simulink library "ssc_Probes_2012a_org"  (Simulink 10.0)
settings: Solver=ode45  StartTime=0.0  StopTime=10.0  RelTol=1e-3  EnableMultiTasking=on
libraries: fl_lib x42, nesl_utility x31, fl_ps_legacy_lib x1
(part 1 of 2)
settings Model: Creator=tegel  LastModifiedBy=bhisma

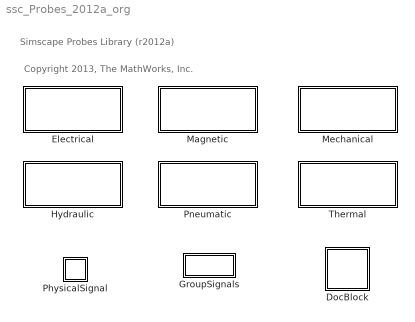
== system ssc_Probes_2012a_org ==
  note: Simscape Probes Library (r2012a)
  note: Copyright 2013, The MathWorks, Inc.
  DocBlock : Subsystem  mask(DocBlock){ECoderFlag=, DocumentType=Text}
      mask prompts: ECoderFlag "RTW Embedded Coder Flag"; DocumentType "Document Type"
      mask help: Use this block to save long descriptive text with the model. Double-clicking the block will open an editor.
      settings: DeleteFcn=docblock('close_document',gcb);  PreSaveFcn=docblock('save_document',gcb);  OpenFcn=docblock('edit_document',gcb);
      mask TypeOptions DocumentType: Text | RTF | HTML
      mask Display: disp('Help')
  Electrical : Subsystem
      mask Display: disp('Electrical')
  GroupSignals : Subsystem
      settings: OpenFcn=GroupSignals
      settings: CopyFcn=|
      | set_param(gcb,'LinkStatus','inactive')
      | set_param(gcb,'LinkStatus','none')
      mask Display: disp('Select')
  Hydraulic : Subsystem
      mask Display: disp('Hydraulic')
  Magnetic : Subsystem
      mask Display: disp('Magnetic');
  Mechanical : Subsystem
      mask Display: disp('Mechanical');
  PhysicalSignal : Subsystem  Description=Simscape Probe  InitFcn=|  StopFcn=|
      InitFcn=|
      | unit=get_param([gcb '/PS-S'],'Unit');                                              
      | set_param(gcb, 'AttributesFormatString', strcat('[', unit,']'));
      StopFcn=|
      | % Convert logsout to Dataset                                
      | if ~strcmp(class(logsout),'Simulink.SimulationData.Dataset')
      | logsout = logsout.convertToDataset('logsout');              
      | end
      mask help: Simscape Probe
      settings: CopyFcn=|
      | set_param(gcb,'LinkStatus','inactive');
      | set_param(gcb,'LinkStatus','none');
      | set_param([gcb '/Goto'],'GotoTag', [get(gcbh,'name')]);
      | set_param([gcb '/From'],'GotoTag', [get(gcbh,'name')]);
      | h = get_param([gcb, '/PS-S'], 'PortHandles');
      | set(h.Outport(1), 'SignalNameFromLabel', [get(gcbh,'name')])
      | clear h;
      settings: NameChangeFcn=|
      | set_param([gcb '/Goto'],'GotoTag', [get(gcbh,'name')]);
      | set_param([gcb '/From'],'GotoTag', [get(gcbh,'name')]);
      | h = get_param([gcb, '/PS-S'], 'PortHandles');
      | set(h.Outport(1), 'SignalNameFromLabel', [get(gcbh,'name')])
      | clear h;
      settings: OpenFcn=|
      | if exist('logsout', 'var')
      |   vname = get(gcbh,'name');
      |   fHandle = findall(0,'Tag',vname);
      |   if isempty(fHandle)
      |   figure('Tag',vname);
      |   end;
      |   figure(findobj('Tag',vname));
      |   plot(logsout.getElement([gcb, '/PS-S'], '-blockpath').Values)
      |   title(get(gcbh,'name'));
      |   ylabel(['Physical Signal (' get_param([gcb '/PS-S'],'Unit') ')'] );
      | end
      mask Display: disp('PS');
  Pneumatic : Subsystem
      mask Display: disp('Pneumatic');
  Thermal : Subsystem
      mask Display: disp('Thermal');

== system ssc_Probes_2012a_org/DocBlock ==
  EmptySubsystem : Subsystem

== system ssc_Probes_2012a_org/Electrical ==
  note: Electrical Probes
  note: Across Variable
      | (Internal Reference)
  note: Through
      | Variable
  note: Across Variable
      | (Differential)
  Current : Subsystem  Description=Simscape Probe  InitFcn=|  StopFcn=|
      InitFcn=|
      | unit=get_param([gcb '/PS-S'],'Unit');                                              
      | set_param(gcb, 'AttributesFormatString', strcat('[', unit,']'));
      StopFcn=|
      | % Convert logsout to Dataset                                
      | if ~strcmp(class(logsout),'Simulink.SimulationData.Dataset')
      | logsout = logsout.convertToDataset('logsout');              
      | end
      mask help: Simscape Probe
      settings: CopyFcn=|
      | set_param(gcb,'LinkStatus','inactive');
      | set_param(gcb,'LinkStatus','none');
      | set_param([gcb '/Goto'],'GotoTag', [get(gcbh,'name')]);
      | set_param([gcb '/From'],'GotoTag', [get(gcbh,'name')]);
      | h = get_param([gcb, '/PS-S'], 'PortHandles');
      | set(h.Outport(1), 'SignalNameFromLabel', [get(gcbh,'name')])
      | clear h;
      settings: NameChangeFcn=|
      | set_param([gcb '/Goto'],'GotoTag', [get(gcbh,'name')]);
      | set_param([gcb '/From'],'GotoTag', [get(gcbh,'name')]);
      | h = get_param([gcb, '/PS-S'], 'PortHandles');
      | set(h.Outport(1), 'SignalNameFromLabel', [get(gcbh,'name')])
      | clear h;
      settings: OpenFcn=|
      | if exist('logsout', 'var')
      |   vname = get(gcbh,'name');
      |   fHandle = findall(0,'Tag',vname);
      |   if isempty(fHandle)
      |   figure('Tag',vname);
      |   end;
      |   figure(findobj('Tag',vname));
      |   plot(logsout.getElement([gcb, '/PS-S'], '-blockpath').Values)
      |   title(get(gcbh,'name'));
      |   ylabel(['Current (' get_param([gcb '/PS-S'],'Unit') ')'] );
      | end
      mask Display:
      | patch([0.5 1 0.5], [0.25 .5 0.75],[0.7 0.7 0.7])
      | plot([0,0.5],[0.5,0.5]);
  Voltage : Subsystem  Description=Simscape Probe  InitFcn=|  StopFcn=|
      InitFcn=|
      | unit=get_param([gcb '/PS-S'],'Unit');                                              
      | set_param(gcb, 'AttributesFormatString', strcat('[', unit,']'));
      StopFcn=|
      | % Convert logsout to Dataset                                
      | if ~strcmp(class(logsout),'Simulink.SimulationData.Dataset')
      | logsout = logsout.convertToDataset('logsout');              
      | end
      mask help: Simscape Probe
      settings: CopyFcn=|
      | set_param(gcb,'LinkStatus','inactive');
      | set_param(gcb,'LinkStatus','none');
      | set_param([gcb '/Goto'],'GotoTag', [get(gcbh,'name')]);
      | set_param([gcb '/From'],'GotoTag', [get(gcbh,'name')]);
      | h = get_param([gcb, '/PS-S'], 'PortHandles');
      | set(h.Outport(1), 'SignalNameFromLabel', [get(gcbh,'name')])
      | clear h;
      settings: NameChangeFcn=|
      | set_param([gcb '/Goto'],'GotoTag', [get(gcbh,'name')]);
      | set_param([gcb '/From'],'GotoTag', [get(gcbh,'name')]);
      | h = get_param([gcb, '/PS-S'], 'PortHandles');
      | set(h.Outport(1), 'SignalNameFromLabel', [get(gcbh,'name')])
      | clear h;
      settings: OpenFcn=|
      | if exist('logsout', 'var')
      |   vname = get(gcbh,'name');
      |   fHandle = findall(0,'Tag',vname);
      |   if isempty(fHandle)
      |   figure('Tag',vname);
      |   end;
      |   figure(findobj('Tag',vname));
      |   plot(logsout.getElement([gcb, '/PS-S'], '-blockpath').Values)
      |   title(get(gcbh,'name'));
      |   ylabel(['Voltage (' get_param([gcb '/PS-S'],'Unit') ')'] );
      | end
      mask Display: port_label('LConn', 1,'V');
  dVoltage : Subsystem  Description=Simscape Probe  InitFcn=|  StopFcn=|
      InitFcn=|
      | unit=get_param([gcb '/PS-S'],'Unit');                                              
      | set_param(gcb, 'AttributesFormatString', strcat('[', unit,']'));
      StopFcn=|
      | % Convert logsout to Dataset                                
      | if ~strcmp(class(logsout),'Simulink.SimulationData.Dataset')
      | logsout = logsout.convertToDataset('logsout');              
      | end
      mask help: Simscape Probe
      settings: CopyFcn=|
      | set_param(gcb,'LinkStatus','inactive');
      | set_param(gcb,'LinkStatus','none');
      | set_param([gcb '/Goto'],'GotoTag', [get(gcbh,'name')]);
      | set_param([gcb '/From'],'GotoTag', [get(gcbh,'name')]);
      | h = get_param([gcb, '/PS-S'], 'PortHandles');
      | set(h.Outport(1), 'SignalNameFromLabel', [get(gcbh,'name')])
      | clear h;
      settings: NameChangeFcn=|
      | set_param([gcb '/Goto'],'GotoTag', [get(gcbh,'name')]);
      | set_param([gcb '/From'],'GotoTag', [get(gcbh,'name')]);
      | h = get_param([gcb, '/PS-S'], 'PortHandles');
      | set(h.Outport(1), 'SignalNameFromLabel', [get(gcbh,'name')])
      | clear h;
      settings: OpenFcn=|
      | if exist('logsout', 'var')
      |   vname = get(gcbh,'name');
      |   fHandle = findall(0,'Tag',vname);
      |   if isempty(fHandle)
      |   figure('Tag',vname);
      |   end;
      |   figure(findobj('Tag',vname));
      |   plot(logsout.getElement([gcb, '/PS-S'], '-blockpath').Values)
      |   title(get(gcbh,'name'));
      |   ylabel(['Voltage (' get_param([gcb '/PS-S'],'Unit') ')'] );
      | end
      mask Display:
      | port_label('RConn', 1,'-');
      | port_label('LConn', 1,'+');

== system ssc_Probes_2012a_org/GroupSignals ==

== system ssc_Probes_2012a_org/Hydraulic ==
  note: Hydraulic Probes
  note: Across Variable
      | (Internal Reference)
  note: Through
      | Variable
  note: Across Variable
      | (Differential)
  Flow : Subsystem  Description=Simscape Probe  InitFcn=|  StopFcn=|
      InitFcn=|
      | unit=get_param([gcb '/PS-S'],'Unit');                                              
      | set_param(gcb, 'AttributesFormatString', strcat('[', unit,']'));
      StopFcn=|
      | % Convert logsout to Dataset                                
      | if ~strcmp(class(logsout),'Simulink.SimulationData.Dataset')
      | logsout = logsout.convertToDataset('logsout');              
      | end
      mask help: Simscape Probe
      settings: CopyFcn=|
      | set_param(gcb,'LinkStatus','inactive');
      | set_param(gcb,'LinkStatus','none');
      | set_param([gcb '/Goto'],'GotoTag', [get(gcbh,'name')]);
      | set_param([gcb '/From'],'GotoTag', [get(gcbh,'name')]);
      | h = get_param([gcb, '/PS-S'], 'PortHandles');
      | set(h.Outport(1), 'SignalNameFromLabel', [get(gcbh,'name')])
      | clear h;
      settings: NameChangeFcn=|
      | set_param([gcb '/Goto'],'GotoTag', [get(gcbh,'name')]);
      | set_param([gcb '/From'],'GotoTag', [get(gcbh,'name')]);
      | h = get_param([gcb, '/PS-S'], 'PortHandles');
      | set(h.Outport(1), 'SignalNameFromLabel', [get(gcbh,'name')])
      | clear h;
      settings: OpenFcn=|
      | if exist('logsout', 'var')
      |   vname = get(gcbh,'name');
      |   fHandle = findall(0,'Tag',vname);
      |   if isempty(fHandle)
      |   figure('Tag',vname);
      |   end;
      |   figure(findobj('Tag',vname));
      |   plot(logsout.getElement([gcb, '/PS-S'], '-blockpath').Values)
      |   title(get(gcbh,'name'));
      |   ylabel(['Flow (' get_param([gcb '/PS-S'],'Unit') ')'] );
      | end
      mask Display:
      | patch([0.5 1 0.5], [0.25 .5 0.75],[0.7 0.7 0.7])
      | plot([0,0.5],[0.5,0.5]);
  Pressure : Subsystem  Description=Simscape Probe  InitFcn=|  StopFcn=|
      InitFcn=|
      | unit=get_param([gcb '/PS-S'],'Unit');                                              
      | set_param(gcb, 'AttributesFormatString', strcat('[', unit,']'));
      StopFcn=|
      | % Convert logsout to Dataset                                
      | if ~strcmp(class(logsout),'Simulink.SimulationData.Dataset')
      | logsout = logsout.convertToDataset('logsout');              
      | end
      mask help: Simscape Probe
      settings: CopyFcn=|
      | set_param(gcb,'LinkStatus','inactive');
      | set_param(gcb,'LinkStatus','none');
      | set_param([gcb '/Goto'],'GotoTag', [get(gcbh,'name')]);
      | set_param([gcb '/From'],'GotoTag', [get(gcbh,'name')]);
      | h = get_param([gcb, '/PS-S'], 'PortHandles');
      | set(h.Outport(1), 'SignalNameFromLabel', [get(gcbh,'name')])
      | clear h;
      settings: NameChangeFcn=|
      | set_param([gcb '/Goto'],'GotoTag', [get(gcbh,'name')]);
      | set_param([gcb '/From'],'GotoTag', [get(gcbh,'name')]);
      | h = get_param([gcb, '/PS-S'], 'PortHandles');
      | set(h.Outport(1), 'SignalNameFromLabel', [get(gcbh,'name')])
      | clear h;
      settings: OpenFcn=|
      | if exist('logsout', 'var')
      |   vname = get(gcbh,'name');
      |   fHandle = findall(0,'Tag',vname);
      |   if isempty(fHandle)
      |   figure('Tag',vname);
      |   end;
      |   figure(findobj('Tag',vname));
      |   plot(logsout.getElement([gcb, '/PS-S'], '-blockpath').Values)
      |   title(get(gcbh,'name'));
      |   ylabel(['Pressure (' get_param([gcb '/PS-S'],'Unit') ')'] );
      | end
      mask Display: port_label('LConn', 1,'P');
  dPressure : Subsystem  Description=Simscape Probe  InitFcn=|  StopFcn=|
      InitFcn=|
      | unit=get_param([gcb '/PS-S'],'Unit');                                             
      | set_param(gcb, 'AttributesFormatString', strcat('[', unit,']'));
      StopFcn=|
      | % Convert logsout to Dataset                                
      | if ~strcmp(class(logsout),'Simulink.SimulationData.Dataset')
      | logsout = logsout.convertToDataset('logsout');              
      | end
      mask help: Simscape Probe
      settings: CopyFcn=|
      | set_param(gcb,'LinkStatus','inactive');
      | set_param(gcb,'LinkStatus','none');
      | set_param([gcb '/Goto'],'GotoTag', [get(gcbh,'name')]);
      | set_param([gcb '/From'],'GotoTag', [get(gcbh,'name')]);
      | h = get_param([gcb, '/PS-S'], 'PortHandles');
      | set(h.Outport(1), 'SignalNameFromLabel', [get(gcbh,'name')])
      | clear h;
      settings: NameChangeFcn=|
      | set_param([gcb '/Goto'],'GotoTag', [get(gcbh,'name')]);
      | set_param([gcb '/From'],'GotoTag', [get(gcbh,'name')]);
      | h = get_param([gcb, '/PS-S'], 'PortHandles');
      | set(h.Outport(1), 'SignalNameFromLabel', [get(gcbh,'name')])
      | clear h;
      settings: OpenFcn=|
      | if exist('logsout', 'var')
      |   vname = get(gcbh,'name');
      |   fHandle = findall(0,'Tag',vname);
      |   if isempty(fHandle)
      |   figure('Tag',vname);
      |   end;
      |   figure(findobj('Tag',vname));
      |   plot(logsout.getElement([gcb, '/PS-S'], '-blockpath').Values)
      |   title(get(gcbh,'name'));
      |   ylabel(['Pressure (' get_param([gcb '/PS-S'],'Unit') ')'] );
      | end
      mask Display:
      | port_label('RConn', 1,'-');
      | port_label('LConn', 1,'+');

== system ssc_Probes_2012a_org/Magnetic ==
  note: Across Variable
      | (Differential)
  note: Through
      | Variable
  note: Across Variable
      | (Internal Reference)
  note: MagneticProbes
  Flux : Subsystem  Description=Simscape Probe  InitFcn=|  StopFcn=|
      InitFcn=|
      | unit=get_param([gcb '/PS-S'],'Unit');                                              
      | set_param(gcb, 'AttributesFormatString', strcat('[', unit,']'));
      StopFcn=|
      | % Convert logsout to Dataset                                
      | if ~strcmp(class(logsout),'Simulink.SimulationData.Dataset')
      | logsout = logsout.convertToDataset('logsout');              
      | end
      mask help: Simscape Probe
      settings: CopyFcn=|
      | set_param(gcb,'LinkStatus','inactive');
      | set_param(gcb,'LinkStatus','none');
      | set_param([gcb '/Goto'],'GotoTag', [get(gcbh,'name')]);
      | set_param([gcb '/From'],'GotoTag', [get(gcbh,'name')]);
      | h = get_param([gcb, '/PS-S'], 'PortHandles');
      | set(h.Outport(1), 'SignalNameFromLabel', [get(gcbh,'name')])
      | clear h;
      settings: NameChangeFcn=|
      | set_param([gcb '/Goto'],'GotoTag', [get(gcbh,'name')]);
      | set_param([gcb '/From'],'GotoTag', [get(gcbh,'name')]);
      | h = get_param([gcb, '/PS-S'], 'PortHandles');
      | set(h.Outport(1), 'SignalNameFromLabel', [get(gcbh,'name')])
      | clear h;
      settings: OpenFcn=|
      | if exist('logsout', 'var')
      |   vname = get(gcbh,'name');
      |   fHandle = findall(0,'Tag',vname);
      |   if isempty(fHandle)
      |   figure('Tag',vname);
      |   end;
      |   figure(findobj('Tag',vname));
      |   plot(logsout.getElement([gcb, '/PS-S'], '-blockpath').Values)
      |   title(get(gcbh,'name'));
      |   ylabel(['Flux (' get_param([gcb '/PS-S'],'Unit') ')'] );
      | end
      mask Display:
      | patch([0.5 1 0.5], [0.25 .5 0.75],[0.7 0.7 0.7])
      | plot([0,0.5],[0.5,0.5]);
  MMF : Subsystem  Description=Simscape Probe  InitFcn=|  StopFcn=|
      InitFcn=|
      | unit=get_param([gcb '/PS-S'],'Unit');                                              
      | set_param(gcb, 'AttributesFormatString', strcat('[', unit,']'));
      StopFcn=|
      | % Convert logsout to Dataset                                
      | if ~strcmp(class(logsout),'Simulink.SimulationData.Dataset')
      | logsout = logsout.convertToDataset('logsout');              
      | end
      mask help: Simscape Probe
      settings: CopyFcn=|
      | set_param(gcb,'LinkStatus','inactive');
      | set_param(gcb,'LinkStatus','none');
      | set_param([gcb '/Goto'],'GotoTag', [get(gcbh,'name')]);
      | set_param([gcb '/From'],'GotoTag', [get(gcbh,'name')]);
      | h = get_param([gcb, '/PS-S'], 'PortHandles');
      | set(h.Outport(1), 'SignalNameFromLabel', [get(gcbh,'name')])
      | clear h;
      settings: NameChangeFcn=|
      | set_param([gcb '/Goto'],'GotoTag', [get(gcbh,'name')]);
      | set_param([gcb '/From'],'GotoTag', [get(gcbh,'name')]);
      | h = get_param([gcb, '/PS-S'], 'PortHandles');
      | set(h.Outport(1), 'SignalNameFromLabel', [get(gcbh,'name')])
      | clear h;
      settings: OpenFcn=|
      | if exist('logsout', 'var')
      |   vname = get(gcbh,'name');
      |   fHandle = findall(0,'Tag',vname);
      |   if isempty(fHandle)
      |   figure('Tag',vname);
      |   end;
      |   figure(findobj('Tag',vname));
      |   plot(logsout.getElement([gcb, '/PS-S'], '-blockpath').Values)
      |   title(get(gcbh,'name'));
      |   ylabel(['MMF (' get_param([gcb '/PS-S'],'Unit') ')'] );
      | end
      mask Display: port_label('LConn', 1,'F');
  dMMF : Subsystem  Description=Simscape Probe  InitFcn=|  StopFcn=|
      InitFcn=|
      | unit=get_param([gcb '/PS-S'],'Unit');                                              
      | set_param(gcb, 'AttributesFormatString', strcat('[', unit,']'));
      StopFcn=|
      | % Convert logsout to Dataset                                
      | if ~strcmp(class(logsout),'Simulink.SimulationData.Dataset')
      | logsout = logsout.convertToDataset('logsout');              
      | end
      mask help: Simscape Probe
      settings: CopyFcn=|
      | set_param(gcb,'LinkStatus','inactive');
      | set_param(gcb,'LinkStatus','none');
      | set_param([gcb '/Goto'],'GotoTag', [get(gcbh,'name')]);
      | set_param([gcb '/From'],'GotoTag', [get(gcbh,'name')]);
      | h = get_param([gcb, '/PS-S'], 'PortHandles');
      | set(h.Outport(1), 'SignalNameFromLabel', [get(gcbh,'name')])
      | clear h;
      settings: NameChangeFcn=|
      | set_param([gcb '/Goto'],'GotoTag', [get(gcbh,'name')]);
      | set_param([gcb '/From'],'GotoTag', [get(gcbh,'name')]);
      | h = get_param([gcb, '/PS-S'], 'PortHandles');
      | set(h.Outport(1), 'SignalNameFromLabel', [get(gcbh,'name')])
      | clear h;
      settings: OpenFcn=|
      | if exist('logsout', 'var')
      |   vname = get(gcbh,'name');
      |   fHandle = findall(0,'Tag',vname);
      |   if isempty(fHandle)
      |   figure('Tag',vname);
      |   end;
      |   figure(findobj('Tag',vname));
      |   plot(logsout.getElement([gcb, '/PS-S'], '-blockpath').Values)
      |   title(get(gcbh,'name'));
      |   ylabel(['MMF (' get_param([gcb '/PS-S'],'Unit') ')'] );
      | end
      mask Display:
      | port_label('RConn', 1,'-');
      | port_label('LConn', 1,'+');

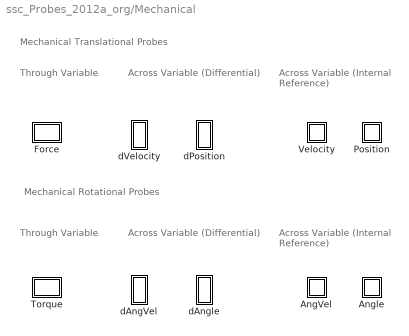
== system ssc_Probes_2012a_org/Mechanical ==
  note: Across Variable
      | (Differential)
  note: Through
      | Variable
  note: Across Variable
      | (Internal Reference)
  note: Mechanical Translational Probes
  note: Across Variable
      | (Differential)
  note: Through
      | Variable
  note: Across Variable
      | (Internal Reference)
  note: Mechanical Rotational Probes
  AngVel : Subsystem  Description=Simscape Probe  InitFcn=|  StopFcn=|
      InitFcn=|
      | unit=get_param([gcb '/PS-S'],'Unit');                                              
      | set_param(gcb, 'AttributesFormatString', strcat('[', unit,']'));
      StopFcn=|
      | % Convert logsout to Dataset                                
      | if ~strcmp(class(logsout),'Simulink.SimulationData.Dataset')
      | logsout = logsout.convertToDataset('logsout');              
      | end
      mask help: Simscape Probe
      settings: CopyFcn=|
      | set_param(gcb,'LinkStatus','inactive');
      | set_param(gcb,'LinkStatus','none');
      | set_param([gcb '/Goto'],'GotoTag', [get(gcbh,'name')]);
      | set_param([gcb '/From'],'GotoTag', [get(gcbh,'name')]);
      | h = get_param([gcb, '/PS-S'], 'PortHandles');
      | set(h.Outport(1), 'SignalNameFromLabel', [get(gcbh,'name')])
      | clear h;
      settings: NameChangeFcn=|
      | set_param([gcb '/Goto'],'GotoTag', [get(gcbh,'name')]);
      | set_param([gcb '/From'],'GotoTag', [get(gcbh,'name')]);
      | h = get_param([gcb, '/PS-S'], 'PortHandles');
      | set(h.Outport(1), 'SignalNameFromLabel', [get(gcbh,'name')])
      | clear h;
      settings: OpenFcn=|
      | if exist('logsout', 'var')
      |   vname = get(gcbh,'name');
      |   fHandle = findall(0,'Tag',vname);
      |   if isempty(fHandle)
      |   figure('Tag',vname);
      |   end;
      |   figure(findobj('Tag',vname));
      |   plot(logsout.getElement([gcb, '/PS-S'], '-blockpath').Values)
      |   title(get(gcbh,'name'));
      |   ylabel(['Anguiar Velocity (' get_param([gcb '/PS-S'],'Unit') ')'] );
      | end
      mask Display: port_label('LConn', 1,'W');
  Angle : Subsystem  Description=Simscape Probe  InitFcn=|  StopFcn=|
      InitFcn=|
      | unit=get_param([gcb '/PS-S'],'Unit');                                              
      | set_param(gcb, 'AttributesFormatString', strcat('[', unit,']'));
      StopFcn=|
      | % Convert logsout to Dataset                                
      | if ~strcmp(class(logsout),'Simulink.SimulationData.Dataset')
      | logsout = logsout.convertToDataset('logsout');              
      | end
      mask help: Simscape Probe
      settings: CopyFcn=|
      | set_param(gcb,'LinkStatus','inactive');
      | set_param(gcb,'LinkStatus','none');
      | set_param([gcb '/Goto'],'GotoTag', [get(gcbh,'name')]);
      | set_param([gcb '/From'],'GotoTag', [get(gcbh,'name')]);
      | h = get_param([gcb, '/PS-S'], 'PortHandles');
      | set(h.Outport(1), 'SignalNameFromLabel', [get(gcbh,'name')])
      | clear h;
      settings: NameChangeFcn=|
      | set_param([gcb '/Goto'],'GotoTag', [get(gcbh,'name')]);
      | set_param([gcb '/From'],'GotoTag', [get(gcbh,'name')]);
      | h = get_param([gcb, '/PS-S'], 'PortHandles');
      | set(h.Outport(1), 'SignalNameFromLabel', [get(gcbh,'name')])
      | clear h;
      settings: OpenFcn=|
      | if exist('logsout', 'var')
      |   vname = get(gcbh,'name');
      |   fHandle = findall(0,'Tag',vname);
      |   if isempty(fHandle)
      |   figure('Tag',vname);
      |   end;
      |   figure(findobj('Tag',vname));
      |   plot(logsout.getElement([gcb, '/PS-S'], '-blockpath').Values)
      |   title(get(gcbh,'name'));
      |   ylabel(['Angle (' get_param([gcb '/PS-S'],'Unit') ')'] );
      | end
      mask Display: port_label('LConn', 1,'A');
  Force : Subsystem  Description=Simscape Probe  InitFcn=|  StopFcn=|
      InitFcn=|
      | unit=get_param([gcb '/PS-S'],'Unit');                                              
      | set_param(gcb, 'AttributesFormatString', strcat('[', unit,']'));
      StopFcn=|
      | % Convert logsout to Dataset                                
      | if ~strcmp(class(logsout),'Simulink.SimulationData.Dataset')
      | logsout = logsout.convertToDataset('logsout');              
      | end
      mask help: Simscape Probe
      settings: CopyFcn=|
      | set_param(gcb,'LinkStatus','inactive');
      | set_param(gcb,'LinkStatus','none');
      | set_param([gcb '/Goto'],'GotoTag', [get(gcbh,'name')]);
      | set_param([gcb '/From'],'GotoTag', [get(gcbh,'name')]);
      | h = get_param([gcb, '/PS-S'], 'PortHandles');
      | set(h.Outport(1), 'SignalNameFromLabel', [get(gcbh,'name')])
      | clear h;
      settings: NameChangeFcn=|
      | set_param([gcb '/Goto'],'GotoTag', [get(gcbh,'name')]);
      | set_param([gcb '/From'],'GotoTag', [get(gcbh,'name')]);
      | h = get_param([gcb, '/PS-S'], 'PortHandles');
      | set(h.Outport(1), 'SignalNameFromLabel', [get(gcbh,'name')])
      | clear h;
      settings: OpenFcn=|
      | if exist('logsout', 'var')
      |   vname = get(gcbh,'name');
      |   fHandle = findall(0,'Tag',vname);
      |   if isempty(fHandle)
      |   figure('Tag',vname);
      |   end;
      |   figure(findobj('Tag',vname));
      |   plot(logsout.getElement([gcb, '/PS-S'], '-blockpath').Values)
      |   title(get(gcbh,'name'));
      |   ylabel(['Force (' get_param([gcb '/PS-S'],'Unit') ')'] );
      | end
      mask Display:
      | patch([0.5 1 0.5], [0.25 .5 0.75],[0.7 0.7 0.7])
      | plot([0,0.5],[0.5,0.5]);
  Position : Subsystem  Description=Simscape Probe  InitFcn=|  StopFcn=|
      InitFcn=|
      | unit=get_param([gcb '/PS-S'],'Unit');                                              
      | set_param(gcb, 'AttributesFormatString', strcat('[', unit,']'));
      StopFcn=|
      | % Convert logsout to Dataset                                
      | if ~strcmp(class(logsout),'Simulink.SimulationData.Dataset')
      | logsout = logsout.convertToDataset('logsout');              
      | end
      mask help: Simscape Probe
      settings: CopyFcn=|
      | set_param(gcb,'LinkStatus','inactive');
      | set_param(gcb,'LinkStatus','none');
      | set_param([gcb '/Goto'],'GotoTag', [get(gcbh,'name')]);
      | set_param([gcb '/From'],'GotoTag', [get(gcbh,'name')]);
      | h = get_param([gcb, '/PS-S'], 'PortHandles');
      | set(h.Outport(1), 'SignalNameFromLabel', [get(gcbh,'name')])
      | clear h;
      settings: NameChangeFcn=|
      | set_param([gcb '/Goto'],'GotoTag', [get(gcbh,'name')]);
      | set_param([gcb '/From'],'GotoTag', [get(gcbh,'name')]);
      | h = get_param([gcb, '/PS-S'], 'PortHandles');
      | set(h.Outport(1), 'SignalNameFromLabel', [get(gcbh,'name')])
      | clear h;
      settings: OpenFcn=|
      | if exist('logsout', 'var')
      |   vname = get(gcbh,'name');
      |   fHandle = findall(0,'Tag',vname);
      |   if isempty(fHandle)
      |   figure('Tag',vname);
      |   end;
      |   figure(findobj('Tag',vname));
      |   plot(logsout.getElement([gcb, '/PS-S'], '-blockpath').Values)
      |   title(get(gcbh,'name'));
      |   ylabel(['Position (' get_param([gcb '/PS-S'],'Unit') ')'] );
      | end
      mask Display: port_label('LConn', 1,'P');
  Torque : Subsystem  Description=Simscape Probe  InitFcn=|  StopFcn=|
      InitFcn=|
      | unit=get_param([gcb '/PS-S'],'Unit');                                              
      | set_param(gcb, 'AttributesFormatString', strcat('[', unit,']'));
      StopFcn=|
      | % Convert logsout to Dataset                                
      | if ~strcmp(class(logsout),'Simulink.SimulationData.Dataset')
      | logsout = logsout.convertToDataset('logsout');              
      | end
      mask help: Simscape Probe
      settings: CopyFcn=|
      | set_param(gcb,'LinkStatus','inactive');
      | set_param(gcb,'LinkStatus','none');
      | set_param([gcb '/Goto'],'GotoTag', [get(gcbh,'name')]);
      | set_param([gcb '/From'],'GotoTag', [get(gcbh,'name')]);
      | h = get_param([gcb, '/PS-S'], 'PortHandles');
      | set(h.Outport(1), 'SignalNameFromLabel', [get(gcbh,'name')])
      | clear h;
      settings: NameChangeFcn=|
      | set_param([gcb '/Goto'],'GotoTag', [get(gcbh,'name')]);
      | set_param([gcb '/From'],'GotoTag', [get(gcbh,'name')]);
      | h = get_param([gcb, '/PS-S'], 'PortHandles');
      | set(h.Outport(1), 'SignalNameFromLabel', [get(gcbh,'name')])
      | clear h;
      settings: OpenFcn=|
      | if exist('logsout', 'var')
      |   vname = get(gcbh,'name');
      |   fHandle = findall(0,'Tag',vname);
      |   if isempty(fHandle)
      |   figure('Tag',vname);
      |   end;
      |   figure(findobj('Tag',vname));
      |   plot(logsout.getElement([gcb, '/PS-S'], '-blockpath').Values)
      |   title(get(gcbh,'name'));
      |   ylabel(['Torque (' get_param([gcb '/PS-S'],'Unit') ')'] );
      | end
      mask Display:
      | patch([0.5 1 0.5], [0.25 .5 0.75],[0.7 0.7 0.7])
      | plot([0,0.5],[0.5,0.5]);
  Velocity : Subsystem  Description=Simscape Probe  InitFcn=|  StopFcn=|
      InitFcn=|
      | unit=get_param([gcb '/PS-S'],'Unit');                                              
      | set_param(gcb, 'AttributesFormatString', strcat('[', unit,']'));
      StopFcn=|
      | % Convert logsout to Dataset                                
      | if ~strcmp(class(logsout),'Simulink.SimulationData.Dataset')
      | logsout = logsout.convertToDataset('logsout');              
      | end
      mask help: Simscape Probe
      settings: CopyFcn=|
      | set_param(gcb,'LinkStatus','inactive');
      | set_param(gcb,'LinkStatus','none');
      | set_param([gcb '/Goto'],'GotoTag', [get(gcbh,'name')]);
      | set_param([gcb '/From'],'GotoTag', [get(gcbh,'name')]);
      | h = get_param([gcb, '/PS-S'], 'PortHandles');
      | set(h.Outport(1), 'SignalNameFromLabel', [get(gcbh,'name')])
      | clear h;
      settings: NameChangeFcn=|
      | set_param([gcb '/Goto'],'GotoTag', [get(gcbh,'name')]);
      | set_param([gcb '/From'],'GotoTag', [get(gcbh,'name')]);
      | h = get_param([gcb, '/PS-S'], 'PortHandles');
      | set(h.Outport(1), 'SignalNameFromLabel', [get(gcbh,'name')])
      | clear h;
      settings: OpenFcn=|
      | if exist('logsout', 'var')
      |   vname = get(gcbh,'name');
      |   fHandle = findall(0,'Tag',vname);
      |   if isempty(fHandle)
      |   figure('Tag',vname);
      |   end;
      |   figure(findobj('Tag',vname));
      |   plot(logsout.getElement([gcb, '/PS-S'], '-blockpath').Values)
      |   title(get(gcbh,'name'));
      |   ylabel(['Velocity (' get_param([gcb '/PS-S'],'Unit') ')'] );
      | end
      mask Display: port_label('LConn', 1,'V');
  dAngVel : Subsystem  Description=Simscape Probe  InitFcn=|  StopFcn=|
      InitFcn=|
      | unit=get_param([gcb '/PS-S'],'Unit');                                              
      | set_param(gcb, 'AttributesFormatString', strcat('[', unit,']'));
      StopFcn=|
      | % Convert logsout to Dataset                                
      | if ~strcmp(class(logsout),'Simulink.SimulationData.Dataset')
      | logsout = logsout.convertToDataset('logsout');              
      | end
      mask help: Simscape Probe
      settings: CopyFcn=|
      | set_param(gcb,'LinkStatus','inactive');
      | set_param(gcb,'LinkStatus','none');
      | set_param([gcb '/Goto'],'GotoTag', [get(gcbh,'name')]);
      | set_param([gcb '/From'],'GotoTag', [get(gcbh,'name')]);
      | h = get_param([gcb, '/PS-S'], 'PortHandles');
      | set(h.Outport(1), 'SignalNameFromLabel', [get(gcbh,'name')])
      | clear h;
      settings: NameChangeFcn=|
      | set_param([gcb '/Goto'],'GotoTag', [get(gcbh,'name')]);
      | set_param([gcb '/From'],'GotoTag', [get(gcbh,'name')]);
      | h = get_param([gcb, '/PS-S'], 'PortHandles');
      | set(h.Outport(1), 'SignalNameFromLabel', [get(gcbh,'name')])
      | clear h;
      settings: OpenFcn=|
      | if exist('logsout', 'var')
      |   vname = get(gcbh,'name');
      |   fHandle = findall(0,'Tag',vname);
      |   if isempty(fHandle)
      |   figure('Tag',vname);
      |   end;
      |   figure(findobj('Tag',vname));
      |   plot(logsout.getElement([gcb, '/PS-S'], '-blockpath').Values)
      |   title(get(gcbh,'name'));
      |   ylabel(['Angular Velocity (' get_param([gcb '/PS-S'],'Unit') ')'] );
      | end
      mask Display:
      | port_label('RConn', 1,'-');
      | port_label('LConn', 1,'+');
  dAngle : Subsystem  Description=Simscape Probe  InitFcn=|  StopFcn=|
      InitFcn=|
      | unit=get_param([gcb '/PS-S'],'Unit');                                              
      | set_param(gcb, 'AttributesFormatString', strcat('[', unit,']'));
      StopFcn=|
      | % Convert logsout to Dataset                                
      | if ~strcmp(class(logsout),'Simulink.SimulationData.Dataset')
      | logsout = logsout.convertToDataset('logsout');              
      | end
      mask help: Simscape Probe
      settings: CopyFcn=|
      | set_param(gcb,'LinkStatus','inactive');
      | set_param(gcb,'LinkStatus','none');
      | set_param([gcb '/Goto'],'GotoTag', [get(gcbh,'name')]);
      | set_param([gcb '/From'],'GotoTag', [get(gcbh,'name')]);
      | h = get_param([gcb, '/PS-S'], 'PortHandles');
      | set(h.Outport(1), 'SignalNameFromLabel', [get(gcbh,'name')])
      | clear h;
      settings: NameChangeFcn=|
      | set_param([gcb '/Goto'],'GotoTag', [get(gcbh,'name')]);
      | set_param([gcb '/From'],'GotoTag', [get(gcbh,'name')]);
      | h = get_param([gcb, '/PS-S'], 'PortHandles');
      | set(h.Outport(1), 'SignalNameFromLabel', [get(gcbh,'name')])
      | clear h;
      settings: OpenFcn=|
      | if exist('logsout', 'var')
      |   vname = get(gcbh,'name');
      |   fHandle = findall(0,'Tag',vname);
      |   if isempty(fHandle)
      |   figure('Tag',vname);
      |   end;
      |   figure(findobj('Tag',vname));
      |   plot(logsout.getElement([gcb, '/PS-S'], '-blockpath').Values)
      |   title(get(gcbh,'name'));
      |   ylabel(['Angle (' get_param([gcb '/PS-S'],'Unit') ')'] );
      | end
      mask Display:
      | port_label('RConn', 1,'-');
      | port_label('LConn', 1,'+');
  dPosition : Subsystem  Description=Simscape Probe  InitFcn=|  StopFcn=|
      InitFcn=|
      | unit=get_param([gcb '/PS-S'],'Unit');                                              
      | set_param(gcb, 'AttributesFormatString', strcat('[', unit,']'));
      StopFcn=|
      | % Convert logsout to Dataset                                
      | if ~strcmp(class(logsout),'Simulink.SimulationData.Dataset')
      | logsout = logsout.convertToDataset('logsout');              
      | end
      mask help: Simscape Probe
      settings: CopyFcn=|
      | set_param(gcb,'LinkStatus','inactive');
      | set_param(gcb,'LinkStatus','none');
      | set_param([gcb '/Goto'],'GotoTag', [get(gcbh,'name')]);
      | set_param([gcb '/From'],'GotoTag', [get(gcbh,'name')]);
      | h = get_param([gcb, '/PS-S'], 'PortHandles');
      | set(h.Outport(1), 'SignalNameFromLabel', [get(gcbh,'name')])
      | clear h;
      settings: NameChangeFcn=|
      | set_param([gcb '/Goto'],'GotoTag', [get(gcbh,'name')]);
      | set_param([gcb '/From'],'GotoTag', [get(gcbh,'name')]);
      | h = get_param([gcb, '/PS-S'], 'PortHandles');
      | set(h.Outport(1), 'SignalNameFromLabel', [get(gcbh,'name')])
      | clear h;
      settings: OpenFcn=|
      | if exist('logsout', 'var')
      |   vname = get(gcbh,'name');
      |   fHandle = findall(0,'Tag',vname);
      |   if isempty(fHandle)
      |   figure('Tag',vname);
      |   end;
      |   figure(findobj('Tag',vname));
      |   plot(logsout.getElement([gcb, '/PS-S'], '-blockpath').Values)
      |   title(get(gcbh,'name'));
      |   ylabel(['Position (' get_param([gcb '/PS-S'],'Unit') ')'] );
      | end
      mask Display:
      | port_label('RConn', 1,'-');
      | port_label('LConn', 1,'+');
  dVelocity : Subsystem  Description=Simscape Probe  InitFcn=|  StopFcn=|
      InitFcn=|
      | unit=get_param([gcb '/PS-S'],'Unit');                                              
      | set_param(gcb, 'AttributesFormatString', strcat('[', unit,']'));
      StopFcn=|
      | % Convert logsout to Dataset                                
      | if ~strcmp(class(logsout),'Simulink.SimulationData.Dataset')
      | logsout = logsout.convertToDataset('logsout');              
      | end
      mask help: Simscape Probe
      settings: CopyFcn=|
      | set_param(gcb,'LinkStatus','inactive');
      | set_param(gcb,'LinkStatus','none');
      | set_param([gcb '/Goto'],'GotoTag', [get(gcbh,'name')]);
      | set_param([gcb '/From'],'GotoTag', [get(gcbh,'name')]);
      | h = get_param([gcb, '/PS-S'], 'PortHandles');
      | set(h.Outport(1), 'SignalNameFromLabel', [get(gcbh,'name')])
      | clear h;
      settings: NameChangeFcn=|
      | set_param([gcb '/Goto'],'GotoTag', [get(gcbh,'name')]);
      | set_param([gcb '/From'],'GotoTag', [get(gcbh,'name')]);
      | h = get_param([gcb, '/PS-S'], 'PortHandles');
      | set(h.Outport(1), 'SignalNameFromLabel', [get(gcbh,'name')])
      | clear h;
      settings: OpenFcn=|
      | if exist('logsout', 'var')
      |   vname = get(gcbh,'name');
      |   fHandle = findall(0,'Tag',vname);
      |   if isempty(fHandle)
      |   figure('Tag',vname);
      |   end;
      |   figure(findobj('Tag',vname));
      |   plot(logsout.getElement([gcb, '/PS-S'], '-blockpath').Values)
      |   title(get(gcbh,'name'));
      |   ylabel(['Velocity (' get_param([gcb '/PS-S'],'Unit') ')'] );
      | end
      mask Display:
      | port_label('RConn', 1,'-');
      | port_label('LConn', 1,'+');

== system ssc_Probes_2012a_org/PhysicalSignal ==
  PS Gain : fl_ps_legacy_lib/Legacy Physical Signals/Functions/PS Gain  gain=1
      settings: SourceProductName=Simscape
  PS-S : nesl_utility/PS-Simulink Converter  PhysicalDomain=network_engine_domain  SubClassName=ps_output  LeftPortType=input  RightPortType=output  PseudoPeriodic=off  Frequencies=[]  Unit=1  AffineConversion=off
  Terminator : Terminator
  PS : PMIOPort  Side=Left
  wires:
  PS-S/1 -> [PhysicalSignal]  "PhysicalSignal"
  [PhysicalSignal] -> Terminator/1
  connections:
  PS Gain/RConn1 -- PS-S/LConn1
  PS Gain/LConn1 -- PS/RConn1
